simulink model "PIDfeedforward"  (R2020b)
settings: Solver=VariableStepAuto  StartTime=0.0  StopTime=1.5  RelTol=1e-3
PreLoadFcn:
  | initModelData
  | trajectoryData
  | controlPID
StartFcn:
  | controlPID
values from neighbouring files (symbols this model uses):
  B = Bm + (Kb*Km)/R    (= 0.0149065789474)    [initModelData.m]
  Jm = 6.1e-4    (= 0.00061)    [initModelData.m]
  Kd = R*(3*w*Jm-B)/Km    [controlPID.m]
  Ki = (Jm*R*w^3)/Km    [controlPID.m]
  Km = 0.105    [initModelData.m]
  Kp = 3*(w^2*Jm*R)/Km    [controlPID.m]
  R = 0.76    [initModelData.m]
  r = 156    [initModelData.m]
settings Model: Creator=esdan  LastModifiedBy=esdan

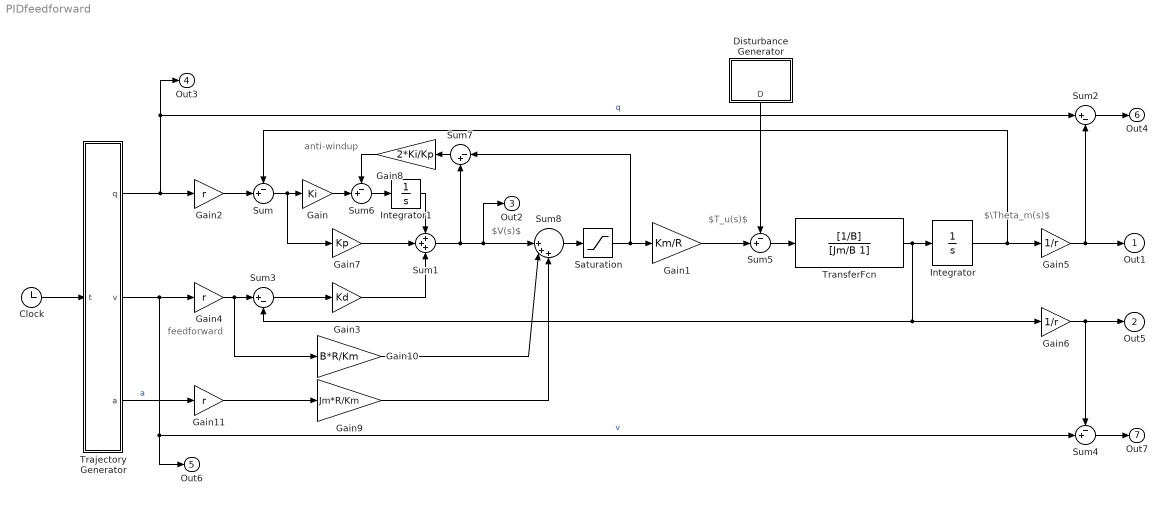
== system PIDfeedforward ==
  note: anti-windup
  note: $\Theta_m(s)$
  note: $V(s)$
  note: $T_u(s)$
  note: feedforward
  Clock : Clock
  Disturbance Generator : Subsystem
  Gain : Gain  Gain=Ki
  Gain1 : Gain  Gain=Km/R
  Gain10 : Gain  Gain=B*R/Km
  Gain11 : Gain  Gain=r
  Gain2 : Gain  Gain=r
  Gain3 : Gain  Gain=Kd
  Gain4 : Gain  Gain=r
  Gain5 : Gain  Gain=1/r
  Gain6 : Gain  Gain=1/r
  Gain7 : Gain  Gain=Kp
  Gain8 : Gain  Gain=2*Ki/Kp
  Gain9 : Gain  Gain=Jm*R/Km
  Integrator : Integrator
  Integrator1 : Integrator
  Saturation : Saturate  UpperLimit=35  LowerLimit=-35
  Sum{,4..6} (4 alike) : Sum  Inputs=-+|
  Sum1 : Sum  Inputs=+++
  Sum2 : Sum  Inputs=|+-
  Sum3 : Sum  Inputs=|+-
  Sum7 : Sum  Inputs=|-+
  Sum8 : Sum  Inputs=||+++
  Trajectory Generator : Subsystem
  TransferFcn : TransferFcn  Numerator=[1/B]  Denominator=[Jm/B 1]
  Out1 : Outport  SignalName=position
  Out5 : Outport  Port=2  SignalName=velocity
  Out2 : Outport  Port=3  SignalName=V
  Out3 : Outport  Port=4  SignalName=position_ref
  Out6 : Outport  Port=5  SignalName=velocity_ref
  Out4 : Outport  Port=6  SignalName=error_position
  Out7 : Outport  Port=7  SignalName=error_velocity
  wires:
  TransferFcn/1 -> Gain6/1, Sum3/2, Integrator/1
  Saturation/1 -> Sum7/1, Gain1/1
  Clock/1 -> Trajectory Generator/1(t)
  Sum/1 -> Gain7/1, Gain/1
  Sum1/1 -> Out2/1, Sum8/1, Sum7/2
  Gain2/1 -> Sum/2
  Trajectory Generator/1(q) -> Gain2/1, Sum2/1, Out3/1  "q"
  Sum2/1 -> Out4/1
  Sum3/1 -> Gain3/1
  Gain5/1 -> Sum2/2, Out1/1
  Integrator/1 -> Gain5/1, Sum/1
  Trajectory Generator/2(v) -> Out6/1, Sum4/2, Gain4/1  "v"
  Gain4/1 -> Gain10/1, Sum3/1
  Gain6/1 -> Out5/1, Sum4/1
  Sum4/1 -> Out7/1
  Sum5/1 -> TransferFcn/1
  Gain1/1 -> Sum5/2
  Disturbance Generator/1(D) -> Sum5/1
  Gain3/1 -> Sum1/3
  Gain7/1 -> Sum1/2
  Gain/1 -> Sum6/2
  Sum7/1 -> Gain8/1
  Gain8/1 -> Sum6/1
  Sum6/1 -> Integrator1/1
  Integrator1/1 -> Sum1/1
  Sum8/1 -> Saturation/1
  Trajectory Generator/3(a) -> Gain11/1  "a"
  Gain11/1 -> Gain9/1
  Gain9/1 -> Sum8/3
  Gain10/1 -> Sum8/2

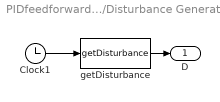
== system PIDfeedforward/Disturbance Generator ==
  Clock1 : Clock
  getDisturbance : MATLABFcn  MATLABFcn=getDisturbance
  D : Outport
  wires:
  Clock1/1 -> getDisturbance/1
  getDisturbance/1 -> D/1

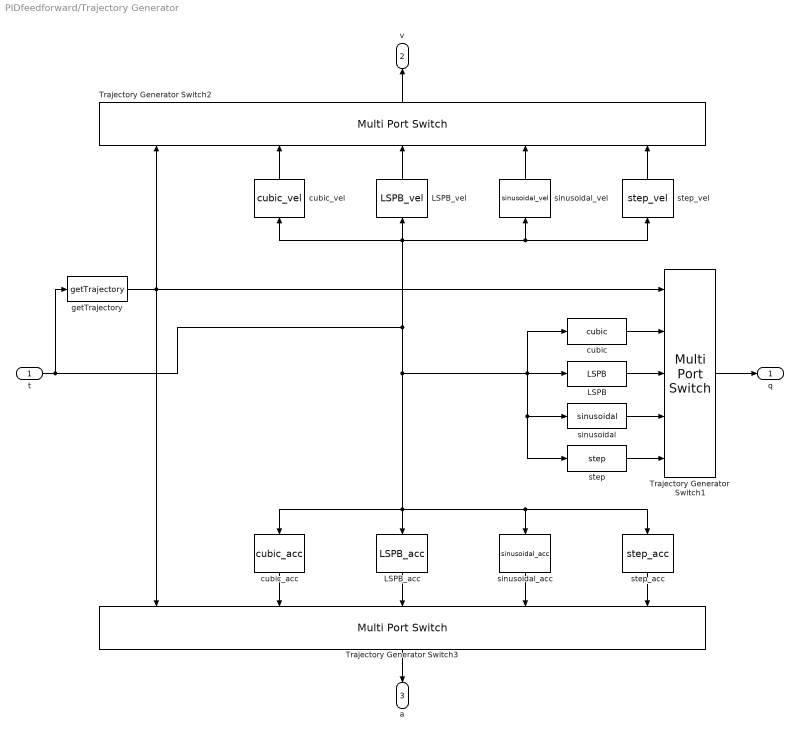
== system PIDfeedforward/Trajectory Generator ==
  t : Inport
  LSPB : MATLABFcn  MATLABFcn=LSPB
  LSPB_acc : MATLABFcn  MATLABFcn=LSPB_acc
  LSPB_vel : MATLABFcn  MATLABFcn=LSPB_vel
  Trajectory Generator Switch1 : MultiPortSwitch  DataPortOrder=Specify indices  Inputs=4  DataPortIndices={CUBIC_,LSPB_,SINUSOIDAL_,STEP_}
  Trajectory Generator Switch2 : MultiPortSwitch  DataPortOrder=Specify indices  Inputs=4  DataPortIndices={CUBIC_,LSPB_,SINUSOIDAL_,STEP_}
  Trajectory Generator Switch3 : MultiPortSwitch  DataPortOrder=Specify indices  Inputs=4  DataPortIndices={CUBIC_,LSPB_,SINUSOIDAL_,STEP_}
  cubic : MATLABFcn  MATLABFcn=cubic
  cubic_acc : MATLABFcn  MATLABFcn=cubic_acc
  cubic_vel : MATLABFcn  MATLABFcn=cubic_vel
  getTrajectory : MATLABFcn  MATLABFcn=getTrajectory
  sinusoidal : MATLABFcn  MATLABFcn=sinusoidal
  sinusoidal_acc : MATLABFcn  MATLABFcn=sinusoidal_acc
  sinusoidal_vel : MATLABFcn  MATLABFcn=sinusoidal_vel
  step : MATLABFcn  MATLABFcn=step
  step_acc : MATLABFcn  MATLABFcn=step_acc
  step_vel : MATLABFcn  MATLABFcn=step_vel
  q : Outport
  v : Outport  Port=2
  a : Outport  Port=3
  wires:
  getTrajectory/1 -> Trajectory Generator Switch3/1, Trajectory Generator Switch1/1, Trajectory Generator Switch2/1
  Trajectory Generator Switch1/1 -> q/1
  step_vel/1 -> Trajectory Generator Switch2/5
  sinusoidal_vel/1 -> Trajectory Generator Switch2/4
  LSPB_vel/1 -> Trajectory Generator Switch2/3
  cubic_vel/1 -> Trajectory Generator Switch2/2
  t/1 -> step_acc/1, sinusoidal_acc/1, cubic_acc/1, LSPB_acc/1, sinusoidal/1, step/1, cubic/1, LSPB/1, sinusoidal_vel/1, step_vel/1, cubic_vel/1, LSPB_vel/1, getTrajectory/1
  Trajectory Generator Switch2/1 -> v/1
  step/1 -> Trajectory Generator Switch1/5
  sinusoidal/1 -> Trajectory Generator Switch1/4
  LSPB/1 -> Trajectory Generator Switch1/3
  cubic/1 -> Trajectory Generator Switch1/2
  step_acc/1 -> Trajectory Generator Switch3/5
  LSPB_acc/1 -> Trajectory Generator Switch3/3
  sinusoidal_acc/1 -> Trajectory Generator Switch3/4
  Trajectory Generator Switch3/1 -> a/1
  cubic_acc/1 -> Trajectory Generator Switch3/2
